simulink model "SDLMackeyGlass"  (R2020b)
settings: Solver=VariableStepAuto  StartTime=0.0  StopTime=config.TFinal  FixedStep=0.01  RelTol=0.01
undefined symbols (not defined in the file): config
settings Model: Creator=tian  LastModifiedBy=tian

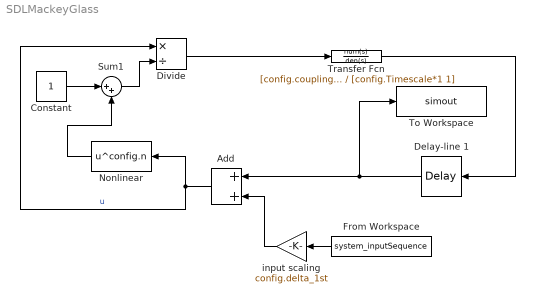
== system SDLMackeyGlass ==
  " Delay-line 1" : TransportDelay  DelayTime=config.tau_a
  Add : Sum
  Constant : Constant
  Divide : Product  Inputs=*/
  From Workspace : FromWorkspace  VariableName=system_inputSequence  SampleTime=config.theta
  Nonlinear : Fcn  Expr=u^config.n
  Sum1 : Sum  Inputs=|++
  To Workspace : ToWorkspace  VariableName=simout  SampleTime=config.sample_time
  Transfer Fcn : TransferFcn  Numerator=[config.coupling]  Denominator=[config.Timescale*1 1]
      mask Display: fprintf('1/s')
  input scaling : Gain  Gain=config.delta_1st
      mask Display: fprintf("%c", 948)
  wires:
  Sum1/1 -> Divide/2
  Nonlinear/1 -> Sum1/2
  From Workspace/1 -> input scaling/1
  Constant/1 -> Sum1/1
  Add/1 -> Nonlinear/1, Divide/1  "u"
  Transfer Fcn/1 -> " Delay-line 1"/1
  input scaling/1 -> Add/2
  " Delay-line 1"/1 -> To Workspace/1, Add/1
  Divide/1 -> Transfer Fcn/1
